simulink model "HEV"  (R2015a)
settings: Solver=ode23tb  StartTime=0.0  StopTime=318  FixedStep=Ts  MaxStep=Ts  RelTol=1  AbsTol=0.5
InitFcn:
  | Ts = 6e-05;   % time step
  | DriveCycleNumber = 1;
  | beginningSim = 1;
undefined symbols (not defined in the file): drive_block, drive_enginemodel, EngineSpeedPower, FuelConsTable, GasEmisTable, h, Hydride, km, magnitude, Metal, Nickel, rad, s, speed, torque
libraries: powerlib x47, driveline x30, simulink x13, simulink_extras x9, electricdrivelib x3, powerlib_extras x3, aerolibconvert2 x2, DC6DriveInternalModels x1
(part 1 of 3)
settings Model: SimulationMode=accelerator  TunableVars=EngineSpeedPower,FuelConsTable,GasEmisTable,ftp75,nedc  TunableVarsStorageClass=Auto,Auto,Auto,Auto,Auto  TunableVarsTypeQualifier=,,,,  Creator=Elena  LastModifiedBy=Elena
settings SolverCC: MaxConsecutiveMinStep=10000  ZeroCrossControl=DisableAll
settings DataIOCC: SaveCompleteFinalSimState=on  SaveFormat=Dataset
settings OptimizationCC: InlineParams=on
settings DebuggingCC: UnderspecifiedInitializationDetection=Classic  SignalResolutionControl=TryResolveAllWithWarning  SigSpecEnsureSampleTimeMsg=none  FcnCallInpInsideContextMsg=UseLocalSettings
settings SimscapeCC: SimscapeLogSimulationStatistics=on

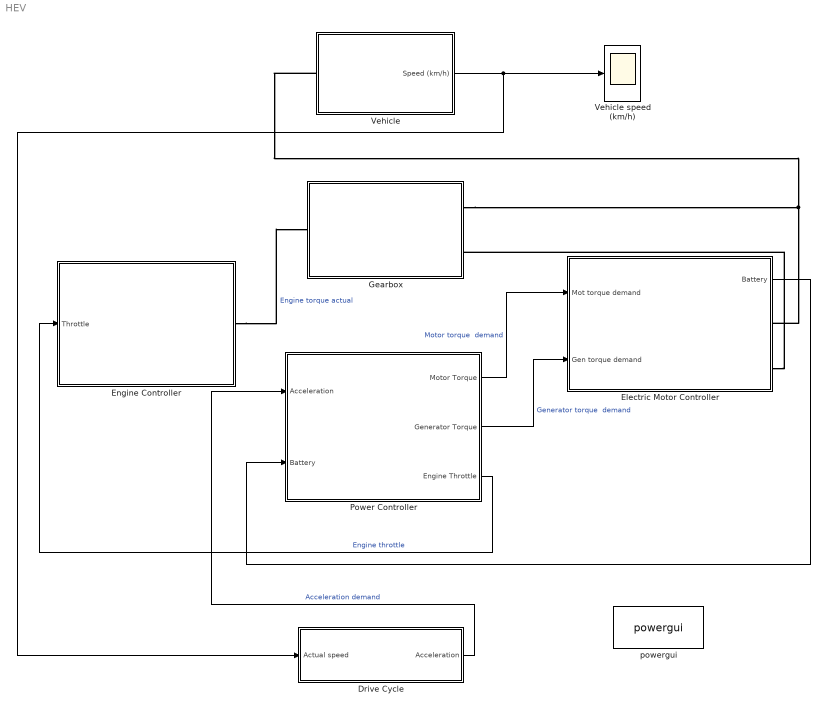
== system HEV ==
  Drive Cycle : Subsystem
  "Electric Motor Controller " : Subsystem
  Engine Controller : Subsystem
  Gearbox : Subsystem
  Power Controller : Subsystem
  Vehicle : Subsystem
  Vehicle speed (km/h) : Scope
      settings: YMin=25.2384  YMax=25.2387  SaveName=ScopeData4  Decimation=10
  powergui : powerlib/powergui  SimulationMode=Discrete  SolverType=Tustin  SampleTime=Ts  frequency=60  SPID=on  DisableSnubberDevices=off  DisableRonSwitches=off  DisableVfSwitches=off  SwTol=0  DisplayEquations=off  Interpol=off  methode=off  Ts=0  FunctionMessages=off  echomessages=off  HookPort=off  EnableUseOfTLC=off  x0status=blocks  frequencyindice=0  Pbase=100e6  ErrMax=1e-4  Iterations=50  UnitsV=kV  UnitsW=MW  buscounter=0  RestoreLinks=warning  ResistiveCurrentMeasurement=off  Frange=[0:2:500]  Ylog=off  Xlog=on  ShowGrid=off  save=off  variable=ZData  structure=0  ZoomFFT=on  StartTime=0.0  cycles=1  DisplayStyle=1  fundamental=60  FreqAxis=off  MaxFrequency=1000  frequencyindicesteady=1  RmsSteady=1  display=off
  wires:
  Power Controller/3(Engine Throttle) -> Engine Controller/1(Throttle)  "Engine throttle"
  Vehicle/1(Speed (km/h)) -> Drive Cycle/1(Actual speed), Vehicle speed (km/h)/1
  Drive Cycle/1("Acceleration ") -> Power Controller/1(Acceleration)  "Acceleration demand"
  "Electric Motor Controller "/1(Battery) -> Power Controller/2(Battery)
  Power Controller/1(Motor Torque) -> "Electric Motor Controller "/1(Mot torque demand)  "Motor torque  demand"
  Power Controller/2(Generator Torque) -> "Electric Motor Controller "/2("Gen torque demand ")  "Generator torque  demand"
  connections:
  Engine Controller/RConn1 -- Gearbox/LConn1  "Engine torque actual"
  Vehicle/LConn1 -- Gearbox/RConn1 -- "Electric Motor Controller "/RConn1
  "Electric Motor Controller "/RConn2 -- Gearbox/RConn2

== system HEV/Drive Cycle ==
  Actual speed : Inport
  Actual speed. : Display
      settings: Decimation=100
  Constant : Constant  Value=final_actualSpeed(end)
  Constant1 : Constant  Value=beginningSim
  Control : Constant  Value=DriveCycleNumber
  Demanded speed : Display
      settings: Decimation=100
  FTP75 : FromWorkspace  VariableName=[ftp75_1.seconds ftp75_1.kph]  SampleTime=0
  Multiport Switch : MultiPortSwitch  Inputs=2
  NEDC : FromWorkspace  VariableName=[nedc.seconds nedc.kph]  SampleTime=0
  Speed Control : Subsystem
  Switch : Switch  Criteria=u2 ~= 0
  To Workspace : ToWorkspace  VariableName=final_actualSpeed  SampleTime=20
      settings: Save2DSignal=2-D array (concatenate along first dimension)
  "Acceleration " : Outport
  wires:
  Control/1 -> Multiport Switch/1
  FTP75/1 -> Multiport Switch/2
  NEDC/1 -> Multiport Switch/3
  Multiport Switch/1 -> Demanded speed/1, Speed Control/1(Demanded speed)
  Speed Control/1(Acceleration) -> "Acceleration "/1
  Constant/1 -> Switch/3
  Actual speed/1 -> Switch/1
  Constant1/1 -> Switch/2
  Switch/1 -> To Workspace/1, Actual speed./1, Speed Control/2(Actual speed)

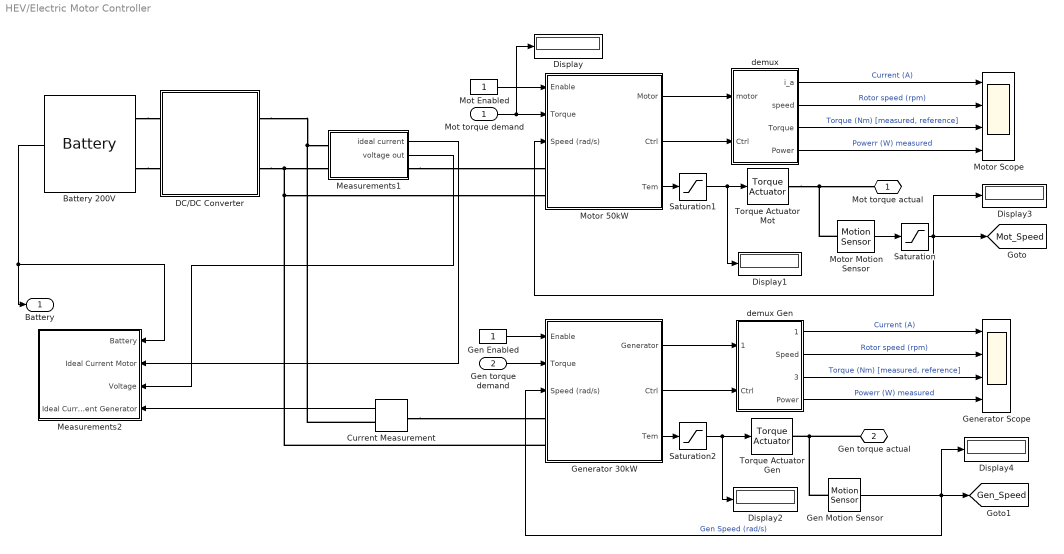
== system HEV/Electric Motor Controller  ==
  Mot torque demand : Inport
  "Gen torque demand " : Inport  Port=2
  Battery 200V : electricdrivelib/Extra Sources/Battery  BatType=Nickel-Metal-Hydride  ShowDetailedParameters=off  NomV=200  NomQ=6.5  SOC=final_SOC(end)  PresetModel=on  MaxQ=7  FullV=235.5932  Dis_rate=1.3  R=0.30769  Normal_OP=6.25  expZone="[216.9492           1.3]"  current=[50 100]  Units=Time  Batt_Tr=30
  Current Measurement : powerlib/Measurements/Current Measurement  PhasorSimulation=off  OutputType=Complex  PSBequivalent=0
  DC/DC Converter : Subsystem
      mask init:
      | [X1,X1m,X2,X2m,X3,X4,Y1,Y1m,Y2,Y2m,Y3,Y4,color1,color2]=spsdrivelogo;
      mask Display:
      | patch([X1 X1m],[Y1 Y1m],color1);
      | patch(X3,Y3,color2);
      | plot([X1 X1m X2 X2m X3 X4],[Y1 Y1m Y2 Y2m Y3 Y4]);
  Display{,1..4} (5 alike) : Display
      settings: Decimation=100
  Gen Enabled : Constant
  Gen Motion Sensor : driveline/Sensors & Actuators/Motion Sensor  Angle=off  x0=0  Velocity=on  Acceleration=off
  Generator 30kW : Subsystem
  Generator Scope : Scope  NumInputPorts=4
      settings: TimeRange=320  YMin=-125~-750~-0.045~-2.5  YMax=125~1500~0.015~1  Decimation=100
  Measurements1 : Subsystem
  Measurements2 : Subsystem
  Mot Enabled : Constant
  Motor 50kW : Subsystem
  Motor Motion Sensor : driveline/Sensors & Actuators/Motion Sensor  Angle=off  x0=0  Velocity=on  Acceleration=off
  Motor Scope : Scope  NumInputPorts=4
      settings: TimeRange=320  YMin=-500~1505.5~-175~3915  YMax=400~1508.25~125~3970  Decimation=100
  Saturation : Saturate  UpperLimit=6000*pi/30  LowerLimit=0
  Saturation1 : Saturate  UpperLimit=400  LowerLimit=-400
  Saturation2 : Saturate  UpperLimit=400  LowerLimit=-400
  Torque Actuator Gen : driveline/Sensors & Actuators/Torque Actuator
  Torque Actuator Mot : driveline/Sensors & Actuators/Torque Actuator
  demux : Subsystem
  demux Gen : Subsystem
  Mot torque actual : PMIOPort  Port=1  Side=Right
  Gen torque actual : PMIOPort  Port=2  Side=Right
  Battery : Outport
  tag scope: Gen_Speed=global, Mot_Speed=global
  wires:
  Battery 200V/1 -> Measurements2/1(Battery), Battery/1
  Mot Enabled/1 -> Motor 50kW/1(Enable)
  Mot torque demand/1 -> Display/1, Motor 50kW/2(Torque)
  "Gen torque demand "/1 -> Generator 30kW/2(Torque)
  Gen Enabled/1 -> Generator 30kW/1(Enable)
  Motor 50kW/1(Motor) -> demux/1(motor)
  Motor 50kW/3(Tem) -> Saturation1/1
  Generator 30kW/3(Tem) -> Saturation2/1
  demux/1(i_a) -> Motor Scope/1  "Current (A)"
  demux/2(speed) -> Motor Scope/2  "Rotor speed (rpm)"
  demux/3(Torque) -> Motor Scope/3  "Torque (Nm) [measured, reference]"
  Generator 30kW/2(Ctrl) -> demux Gen/2(Ctrl)
  Generator 30kW/1(Generator) -> demux Gen/1(Generator)
  demux Gen/1(Current) -> Generator Scope/1  "Current (A)"
  demux Gen/2(Speed) -> Generator Scope/2  "Rotor speed (rpm)"
  demux Gen/3(Torque) -> Generator Scope/3  "Torque (Nm) [measured, reference]"
  demux Gen/4(Power) -> Generator Scope/4  "Powerr (W) measured"
  Measurements1/1(" ideal current ") -> Measurements2/2(Ideal Current Motor)
  Current Measurement/1 -> Measurements2/4(Ideal Current Generator)
  Gen Motion Sensor/1 -> Display4/1, Generator 30kW/3(Speed (rad/s)), [Gen_Speed]  "Gen Speed (rad/s)"
  Motor 50kW/2(Ctrl) -> demux/2(Ctrl)
  Measurements1/2(voltage out) -> Measurements2/3(Voltage)
  Motor Motion Sensor/1 -> Saturation/1
  Saturation1/1 -> Display1/1, Torque Actuator Mot/1
  Saturation2/1 -> Display2/1, Torque Actuator Gen/1
  Saturation/1 -> Display3/1, [Mot_Speed], Motor 50kW/3(Speed (rad/s))
  demux/4(Power) -> Motor Scope/4  "Powerr (W) measured"
  connections:
  Battery 200V/LConn1 -- DC/DC Converter/LConn1
  Battery 200V/LConn2 -- DC/DC Converter/LConn2
  Generator 30kW/LConn2 -- DC/DC Converter/RConn2 -- Measurements1/LConn2 -- Motor 50kW/LConn2
  Current Measurement/RConn1 -- DC/DC Converter/RConn1 -- Measurements1/LConn1
  Measurements1/RConn1 -- Motor 50kW/LConn1
  Current Measurement/LConn1 -- Generator 30kW/LConn1
  Gen torque actual/RConn1 -- Gen Motion Sensor/LConn1 -- Torque Actuator Gen/RConn1
  Torque Actuator Mot/RConn1 -- Motor Motion Sensor/LConn1 -- Mot torque actual/RConn1

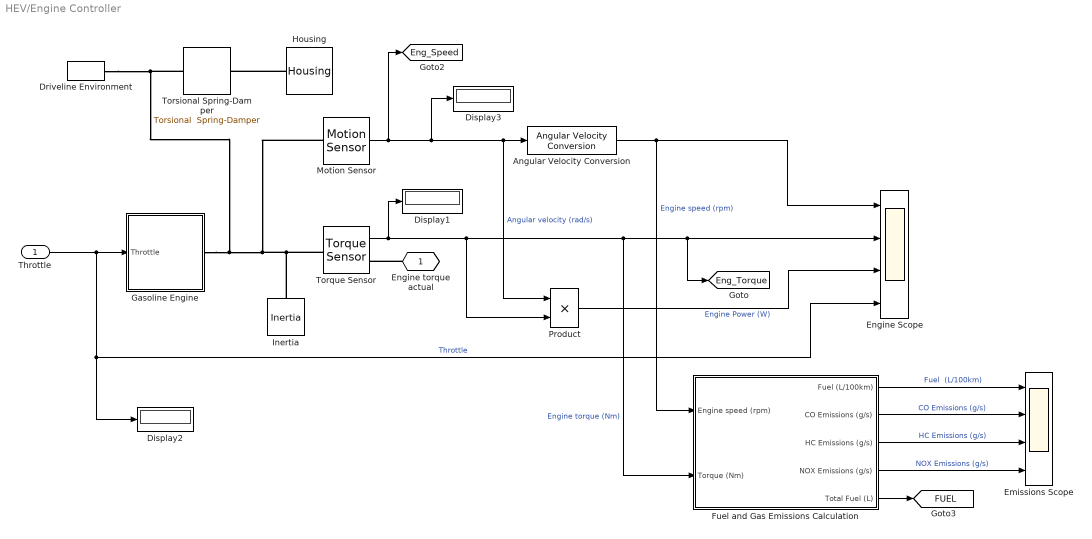
== system HEV/Engine Controller ==
  Throttle : Inport
  Angular Velocity Conversion : aerolibconvert2/Angular Velocity Conversion  IU=rad/s  OU=rpm
  Display1 : Display
      settings: Decimation=100
  Display2 : Display
  Display3 : Display
      settings: Decimation=100
  Driveline Environment : driveline/Solver & Inertias/Driveline Environment  PortType=p1  BlockClass=Solver  PhysicalDomain=driveline_domain  SimulationMode=Dynamics  ModeIteration=on  DefaultClutchVelocityTolerance=1e-3  DefaultUseAutoClutchVelocityTolerance=off
  Emissions Scope : Scope  NumInputPorts=4
      settings: TimeRange=157  YMin=-500~0.187868~0.0455781~-1  YMax=3500~0.187868~0.0455781~1  SaveName=ScopeData5  Decimation=100
  Engine Scope : Scope  NumInputPorts=4
      settings: TimeRange=320  YMin=-500~0~0~-1  YMax=3500~130~800~1  SaveName=ScopeData7  Decimation=100
  Fuel and Gas Emissions Calculation : Subsystem
  Gasoline Engine : Subsystem  AncestorBlock=driveline/Vehicle Components/Gasoline Engine  DialogController=PMDialogs.PMDefaultMaskDlg  LoadFcn=drive_block('LoadFcn');  StartFcn=drive_enginemodel('Start');  mask(Gasoline Engine){power_max=57000, speed_at_power_max=5000, speed_max=6000}
      mask prompts: power_max "Maximum power [W]:"; speed_at_power_max "Speed at maximum power [rpm]:"; speed_max "Maximum speed [rpm]:"
      mask help:
      | Simple gasoline fuel engine model with speed governor.  The throttle input signal lies between zero and one and specifies the torque demanded from the engine as a fraction of the maximum possible torque.  This signal also indirectly controls the engine speed.  The engine model does not include air-fuel combustion dynamics.
      |
      | If the throttle signal rises above one or falls below zero, the engine limits the signal to one or zero, respectively. If the engine speed rises above the maximum speed, the engine torque drops to zero.
      mask init:
      | drive_preinitmask();[speed,power,torque,p] = ...
      | 	drive_enginemodel('MaskGasoline');
      settings: CopyFcn=drive_block('CopyFcn');  DeleteFcn=drive_block('DeleteFcn');  ModelCloseFcn=drive_block('ModelCloseFcn');  PreSaveFcn=drive_block('PreSaveFcn');  PostSaveFcn=drive_block('PostSaveFcn');  PreCopyFcn=drive_block('PreCopyFcn');  PreDeleteFcn=drive_block('PreDeleteFcn');
      mask Help: web(drive_help);
      mask Display:
      | image(imread('engine.bmp'),'center')
      | plot(speed, torque/max(torque))
      | plot(speed, power/max(power))
      | port_label('input', 1, 'Throttle')
  Housing : driveline/Solver & Inertias/Housing
  Inertia : driveline/Solver & Inertias/Inertia  PortType=p1  BlockClass=Inertia  PhysicalDomain=driveline_domain  I=0.25  Ip=[]  Iv=[]  ShowLeft=off  ShowRight=on
  Motion Sensor : driveline/Sensors & Actuators/Motion Sensor  Angle=off  x0=0  Velocity=on  Acceleration=off
  Product : Product
  Torque Sensor : driveline/Sensors & Actuators/Torque Sensor
  Torsional Spring-Damper : driveline/Dynamic Elements/Torsional  Spring-Damper  k=0  c=0.2079  x0=0  Backlash=0
  Engine torque actual : PMIOPort  Port=1  Side=Right
  tag scope: Eng_Speed=global, Eng_Torque=global, FUEL=global
  wires:
  Throttle/1 -> Display2/1, Engine Scope/4, Gasoline Engine/1(Throttle)  "Throttle"
  Motion Sensor/1 -> [Eng_Speed], Display3/1, Angular Velocity Conversion/1, Product/1  "Angular velocity (rad/s)"
  Angular Velocity Conversion/1 -> Fuel and Gas Emissions Calculation/1(Engine speed (rpm)), Engine Scope/1  "Engine speed (rpm)"
  Torque Sensor/1 -> Display1/1, Fuel and Gas Emissions Calculation/2(Torque (Nm)), Engine Scope/2, [Eng_Torque], Product/2  "Engine torque (Nm)"
  Product/1 -> Engine Scope/3  "Engine Power (W)"
  Fuel and Gas Emissions Calculation/1(Fuel (L/100km)) -> Emissions Scope/1  "Fuel  (L/100km)"
  Fuel and Gas Emissions Calculation/2(CO Emissions (g/s)) -> Emissions Scope/2  "CO Emissions (g/s)"
  Fuel and Gas Emissions Calculation/3(HC Emissions (g/s)) -> Emissions Scope/3  "HC Emissions (g/s)"
  Fuel and Gas Emissions Calculation/4(NOX Emissions (g/s)) -> Emissions Scope/4  "NOX Emissions (g/s)"
  Fuel and Gas Emissions Calculation/5(Total Fuel (L)) -> [FUEL]
  connections:
  Motion Sensor/LConn1 -- Driveline Environment/LConn1 -- Torsional Spring-Damper/LConn1 -- Gasoline Engine/RConn1 -- Inertia/RConn1 -- Torque Sensor/LConn1
  Housing/RConn1 -- Torsional Spring-Damper/RConn1
  Engine torque actual/RConn1 -- Torque Sensor/RConn1

== system HEV/Gearbox ==
  Add3 : Sum
  Eng Motion Sensor : driveline/Sensors & Actuators/Motion Sensor  Angle=off  x0=0  Velocity=on  Acceleration=off
  Gen Motion Sensor : driveline/Sensors & Actuators/Motion Sensor  Angle=off  x0=0  Velocity=on  Acceleration=off
  Mot Motion Sensor : driveline/Sensors & Actuators/Motion Sensor  Angle=off  x0=0  Velocity=on  Acceleration=off
  Mux2 : Mux  Inputs=2
  Planetary Gear : driveline/Gears/Planetary Gear  Ratio=2.6  Show=off  LinearizationFlag=off  ValidatorFcn=drive_planetarygearblock
  Power (w) : Scope  NumInputPorts=3
      settings: YMin=-2500~-1000~-2500  YMax=32500~12000~22500  SaveName=ScopeData9  Decimation=100
  Product : Product  RndMeth=Zero
  Product1 : Product  RndMeth=Zero
  Product2 : Product  RndMeth=Zero
  Speed (rad/s) : Scope  NumInputPorts=3
      settings: YMin=5.775e+81~-1.516e+82~-4.5e+68  YMax=6.175e+81~-1.503e+82~5e+67  SaveName=ScopeData3  Decimation=100
  Torque (Nm) : Scope  NumInputPorts=3
      settings: YMin=-10~-5~-2.5  YMax=130~90~35  SaveName=ScopeData10  Decimation=100
  Torque Sensor1 : driveline/Sensors & Actuators/Torque Sensor
  Torque Sensor2 : driveline/Sensors & Actuators/Torque Sensor
  Torque Sensor3 : driveline/Sensors & Actuators/Torque Sensor
  Engine Torque : PMIOPort  Port=1  Side=Left
  Motor Torque : PMIOPort  Port=2  Side=Right
  Generator Torque : PMIOPort  Port=3  Side=Right
  wires:
  Eng Motion Sensor/1 -> Speed (rad/s)/3, Product/1  "Carrier speed (rad/s) - Engine"
  Gen Motion Sensor/1 -> Speed (rad/s)/2, Product2/1  "Sun speed (rad/s) - Generator"
  Mot Motion Sensor/1 -> Speed (rad/s)/1, Product1/2  "Ring speed (rad/s) - Motor"
  Torque Sensor1/1 -> Product/2, Torque (Nm)/1  "Carrier torque (Nm) - Engine"
  Torque Sensor3/1 -> Torque (Nm)/3, Product2/2  "Sun torque (Nm) - Generator"
  Torque Sensor2/1 -> Torque (Nm)/2, Product1/1  "Ring torque (Nm) - Motor"
  Add3/1 -> Mux2/2
  Product/1 -> Mux2/1
  Product1/1 -> Power (w)/3, Add3/1  "Ring power (W) - Motor"
  Product2/1 -> Power (w)/2, Add3/2  "Sun power (W) - Generator"
  Mux2/1 -> Power (w)/1  "Carrier power (W) - Engine"
  connections:
  Torque Sensor2/LConn1 -- Planetary Gear/RConn1
  Eng Motion Sensor/LConn1 -- Planetary Gear/LConn1 -- Torque Sensor1/RConn1
  Torque Sensor1/LConn1 -- Engine Torque/RConn1
  Torque Sensor2/RConn1 -- Mot Motion Sensor/LConn1 -- Motor Torque/RConn1
  Torque Sensor3/RConn1 -- Gen Motion Sensor/LConn1 -- Generator Torque/RConn1
  Torque Sensor3/LConn1 -- Planetary Gear/RConn2

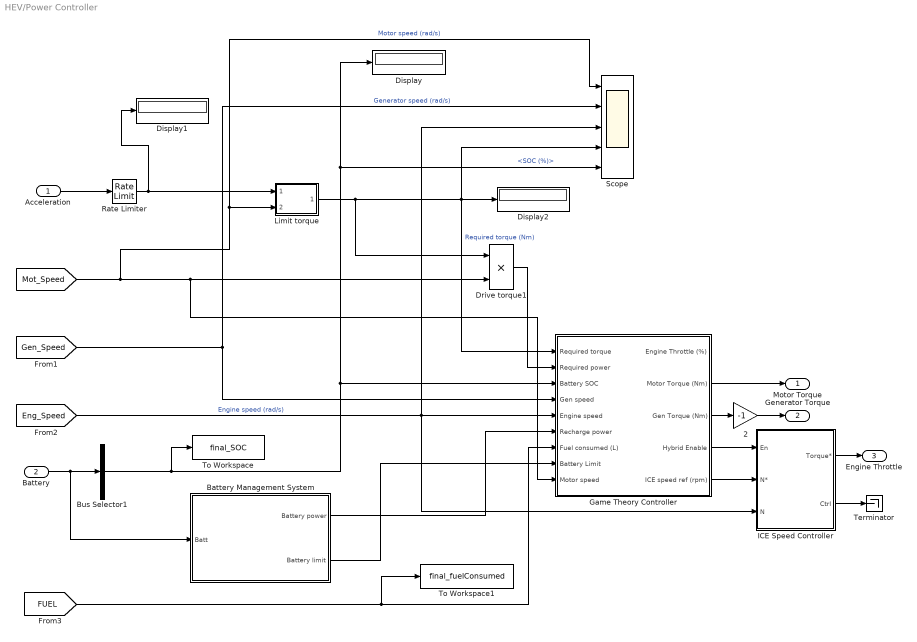
== system HEV/Power Controller ==
  Acceleration : Inport
  Battery : Inport  Port=2
  " 2" : Gain  Gain=-1
  Battery Management System : Subsystem
      mask init:
      | [X1,X1m,X2,X2m,X3,X4,Y1,Y1m,Y2,Y2m,Y3,Y4,color1,color2]=spsdrivelogo;
      mask Display:
      | patch([X1 X1m],[Y1 Y1m],color1);
      | patch(X3,Y3,color2);
      | plot([X1 X1m X2 X2m X3 X4],[Y1 Y1m Y2 Y2m Y3 Y4]);
  Bus Selector1 : BusSelector  OutputSignals=SOC (%)
  Display : Display
      settings: Decimation=100
  Display1 : Display
      settings: Decimation=100
  Display2 : Display
      settings: Decimation=100
  Drive torque1 : Product  Inputs=**  OutDataTypeStr=double
  Game Theory Controller : Subsystem
  ICE Speed Controller : Subsystem  mask(Speed controller){SwK=Speed regulation, bs=1800, ramp=[-5000,5000]*10, kp=0.01, ki=0.1, fc=100, ctrl_sat=[0,1], Tsc=Ts}
      mask prompts: SwK "Regulation type"; bs "Base speed (rpm)"; ramp "Speed reference ramp (rpm/s) [deceleration,acceleration]"; kp "Proportional gain"; ki "Integral gain"; fc "Speed measurement - low-pass filter cutoff frequency (Hz)"; ctrl_sat "Controller output torque saturation (N.m) [negative,positive]"; Tsc "Controller sampling time (s)"
      mask help: This block implements a PI speed regulator.
      mask init:
      | [X1,X1m,X2,X2m,X3,X4,Y1,Y1m,Y2,Y2m,Y3,Y4,color1,color2]=spsdrivelogo;
      mask TypeOptions SwK: Speed regulation | Torque regulation
      mask Display:
      | patch([X1 X1m],[Y1 Y1m],color1);
      | patch(X3,Y3,color2);
      | plot([X1 X1m X2 X2m X3 X4],[Y1 Y1m Y2 Y2m Y3 Y4]);
  Limit torque : Subsystem
      mask Display: plot([0;1800;2000;2500;3000;3500], [1;1;0.90*1;0.72*1;0.6*1;0.51*1])
  Rate Limiter : RateLimiter  SampleTimeMode=inherited
  Scope : Scope  NumInputPorts=5
      settings: TimeRange=318  YMin=0~-750~-50~114~32.5  YMax=350~750~350~122~55  SaveName=ScopeData8  Decimation=100
  Terminator : Terminator
  To Workspace : ToWorkspace  VariableName=final_SOC  SampleTime=20
      settings: Save2DSignal=2-D array (concatenate along first dimension)
  To Workspace1 : ToWorkspace  VariableName=final_fuelConsumed  SampleTime=20
      settings: Save2DSignal=2-D array (concatenate along first dimension)
  Motor Torque : Outport
  Generator Torque : Outport  Port=2
  Engine Throttle : Outport  Port=3
  wires:
  Acceleration/1 -> Rate Limiter/1
  Rate Limiter/1 -> Limit torque/1(Acceleration), Display1/1
  [Mot_Speed] -> Game Theory Controller/9(Motor speed), Drive torque1/2, Limit torque/2(Motor Speed (rad/s)), Scope/1  "Motor speed (rad/s)"
  Limit torque/1(torque) -> Game Theory Controller/1(Required torque), Display2/1, Scope/4, Drive torque1/1  "Required torque (Nm)"
  [Gen_Speed] -> Scope/2, Game Theory Controller/4(Gen speed)  "Generator speed (rad/s)"
  [Eng_Speed] -> Scope/3, Game Theory Controller/5(Engine speed), ICE Speed Controller/3(N)  "Engine speed (rad/s)"
  Game Theory Controller/2(Motor Torque (Nm)) -> Motor Torque/1
  Battery/1 -> Battery Management System/1(Batt), Bus Selector1/1
  Bus Selector1/1 -> To Workspace/1, Display/1, Scope/5, Game Theory Controller/3(Battery SOC)  "<SOC (%)>"
  Battery Management System/1(Battery power) -> Game Theory Controller/6(Recharge power)
  [FUEL] -> To Workspace1/1, Game Theory Controller/7(Fuel consumed (L))
  Drive torque1/1 -> Game Theory Controller/2(Required power)
  Game Theory Controller/3(Gen Torque (Nm)) -> " 2"/1
  " 2"/1 -> Generator Torque/1
  Game Theory Controller/5(ICE speed ref (rpm)) -> ICE Speed Controller/2(N*)
  Game Theory Controller/4(Hybrid Enable) -> ICE Speed Controller/1(En)
  ICE Speed Controller/2(Ctrl) -> Terminator/1
  Battery Management System/2(Battery limit) -> Game Theory Controller/8(Battery Limit)
  ICE Speed Controller/1(Torque*) -> Engine Throttle/1

== system HEV/Vehicle ==
  Differential : driveline/Gears/Differential  R=1  ValidatorFcn=drive_differentialgearblock  SimDrivelineLibraryVersion=1.1
  Display : Display
      settings: Decimation=100
  Housing : driveline/Solver & Inertias/Housing
  Incline angle : Constant  Value=0
  Left Tire : driveline/Vehicle Components/Tire  r_e=0.3  F_z=3000  F_x_max=3500  kappa_max=10  sigma_k=0.2
  Left Tire Inertia : driveline/Solver & Inertias/Inertia  PortType=p1  BlockClass=Inertia  PhysicalDomain=driveline_domain  I=0.5  Ip=[]  Iv=[]  ShowLeft=off  ShowRight=on
  Longitudinal Vehicle Dynamics : driveline/Vehicle Components/Longitudinal Vehicle Dynamics  m=1325  a=1.35  b=1.35  h=0.5  FA=2.57  C_d=0.26  v0=0
  Right Tire : driveline/Vehicle Components/Tire  r_e=0.3  F_z=3000  F_x_max=3500  kappa_max=10  sigma_k=0.2
  Right Tire Inertia : driveline/Solver & Inertias/Inertia  PortType=p1  BlockClass=Inertia  PhysicalDomain=driveline_domain  I=0.5  Ip=[]  Iv=[]  ShowLeft=off  ShowRight=on
  Saturation : Saturate  UpperLimit=200  LowerLimit=0
  Simple Gear : driveline/Gears/Simple Gear  PortType=p1  BlockClass=SimpleGear  PhysicalDomain=driveline_domain  Reversing=off  Ratio=4.113
  Terminator1 : Terminator
  Terminator2 : Terminator
  Torque Sensor : driveline/Sensors & Actuators/Torque Sensor
  Torsional Spring-Damper (Friction) : driveline/Dynamic Elements/Torsional  Spring-Damper  k=0  c=0.1  x0=0  Backlash=0
  Transmission Inertia : driveline/Solver & Inertias/Inertia  PortType=p1  BlockClass=Inertia  PhysicalDomain=driveline_domain  I=0.5  Ip=[]  Iv=[]  ShowLeft=off  ShowRight=on
  m/s to km/h : Gain  Gain=(60*60)/1000
  Torque : PMIOPort  Port=1  Side=Left
  Speed (km/h) : Outport
  tag scope: VehSpeed_kmh=global
  wires:
  Left Tire/2 -> Longitudinal Vehicle Dynamics/1
  Right Tire/2 -> Longitudinal Vehicle Dynamics/2
  Incline angle/1 -> Longitudinal Vehicle Dynamics/3
  Longitudinal Vehicle Dynamics/3 -> Right Tire/2
  Longitudinal Vehicle Dynamics/2 -> Left Tire/2
  Longitudinal Vehicle Dynamics/1 -> m/s to km/h/1, Right Tire/1, Left Tire/1
  Left Tire/1 -> Terminator1/1
  Right Tire/1 -> Terminator2/1
  Torque Sensor/1 -> Display/1
  m/s to km/h/1 -> Saturation/1
  Saturation/1 -> [VehSpeed_kmh], Speed (km/h)/1
  connections:
  Torque Sensor/LConn1 -- Torque/RConn1
  Torsional Spring-Damper (Friction)/RConn1 -- Simple Gear/LConn1 -- Torque Sensor/RConn1
  Housing/RConn1 -- Torsional Spring-Damper (Friction)/LConn1
  Simple Gear/RConn1 -- Transmission Inertia/RConn1 -- Differential/LConn1
  Left Tire Inertia/RConn1 -- Left Tire/LConn1 -- Differential/RConn1
  Right Tire Inertia/RConn1 -- Right Tire/LConn1 -- Differential/RConn2

== system HEV/Drive Cycle/Speed Control ==
  Demanded speed : Inport
  Actual speed : Inport  Port=2
  Display : Display
      settings: Decimation=100
  Display1 : Display
      settings: Decimation=100
  Display2 : Display
      settings: Decimation=100
  Integrator [-5,5] : Integrator  LimitOutput=on  UpperSaturationLimit=5  LowerSaturationLimit=-5
  Ki : Gain  Gain=0.04
  Kp : Gain  Gain=0.02
  Limit : Saturate  UpperLimit=1  LowerLimit=-1
  Lowpass Filter 20Hz : TransferFcn  Denominator=[1/(2*pi*20) 1]
  Mux : Mux  Inputs=2
  Scope : Scope  NumInputPorts=2
      settings: TimeRange=318  YMin=86.25~0.289  YMax=88.75~0.303  SaveName=ScopeData6  Decimation=100
  Sum1 : Sum  Inputs=++|
  Sum2 : Sum  Inputs=+-|
  Acceleration : Outport
  wires:
  Limit/1 -> Display2/1, Acceleration/1, Scope/2  "Acceleration"
  Demanded speed/1 -> Mux/2, Display1/1, Sum2/1  "Demanded speed"
  Actual speed/1 -> Mux/1, Lowpass Filter 20Hz/1  "Actual speed"
  Sum1/1 -> Limit/1
  Ki/1 -> Integrator [-5,5]/1
  Kp/1 -> Sum1/1
  Integrator [-5,5]/1 -> Sum1/2
  Lowpass Filter 20Hz/1 -> Display/1, Sum2/2
  Sum2/1 -> Ki/1, Kp/1
  Mux/1 -> Scope/1  "Speed km/h [actual, reference]"

== system HEV/Electric Motor Controller /DC//DC Converter ==
  Bus DC controller : Subsystem
  DC/DC converter : Subsystem
  Ubus Ref : Constant  Value=500
  +Vdc Bus : PMIOPort  Tag=PMCPort  Port=1  Side=Right
  -Vdc Bus : PMIOPort  Tag=PMCPort  Port=2  Side=Right
  + battery : PMIOPort  Tag=PMCPort  Port=3  Side=Left
  - battery : PMIOPort  Tag=PMCPort  Port=4  Side=Left
  wires:
  Ubus Ref/1 -> Bus DC controller/2(Uref)
  Bus DC controller/1(Duty cycle) -> DC/DC converter/1(Duty Cycle)
  DC/DC converter/1(UBus) -> Bus DC controller/1(Ubus)
  connections:
  +Vdc Bus/RConn1 -- DC/DC converter/LConn1
  -Vdc Bus/RConn1 -- DC/DC converter/LConn2
  + battery/RConn1 -- DC/DC converter/RConn1
  - battery/RConn1 -- DC/DC converter/RConn2

== system HEV/Electric Motor Controller /Generator 30kW ==
  Enable : Inport
  Torque : Inport  Port=2
  Speed (rad/s) : Inport  Port=3
  Bus Selector : BusSelector  OutputSignals=Rotor speed wm (rad/s),Rotor angle thetam (rad),Electromagnetic torque Te (N*m)
  Measures : electricdrivelib/AC drives/PM Synchronous Motor Drive/Measures
  Mux : Subsystem
  PMSM1 : powerlib/Machines/Permanent Magnet Synchronous Machine  NbPhases=3  FluxDistribution=Sinusoidal  RotorType=Salient-pole  MechanicalLoad=Speed w  PresetModel=No  ShowDetailedParameters=on  MeasurementBus=off  Resistance=0.05  Inductance=0  dqInductances=[0.000635 0.000635]  La=0.000835  MachineConstant=Flux linkage established by magnets (V.s)  Flux=0.192  VoltageCst=34.8249  TorqueCst=0.288  Flat=0  Mechanical=[0.011 0.001889/4 4/4]  PolePairs=1  InitialConditions=[0,0, 0,0,0]  InitialConditions5ph=[0 0 0 0 0 0]  TsPowergui=0  TsBlock=-1  RefAngle=90 degrees behind phase A axis (modified Park)
      settings: AttributesFormatString=\n
  Speed Controller : Subsystem  mask(Speed controller){SwK=Torque regulation, bs=1800, ramp=[-5000,5000], kp=(1/5)/4, ki=(50/5)/4/3, fc=(1000/10)/2, ctrl_sat=[-45,45], Tsc=Ts}
      mask prompts: SwK "Regulation type"; bs "Base speed (rpm)"; ramp "Speed reference ramp (rpm/s) [deceleration,acceleration]"; kp "Proportional gain"; ki "Integral gain"; fc "Speed measurement - low-pass filter cutoff frequency (Hz)"; ctrl_sat "Controller output torque saturation (N.m) [negative,positive]"; Tsc "Controller sampling time (s)"
      mask help: This block implements a PI speed regulator.
      mask init:
      | [X1,X1m,X2,X2m,X3,X4,Y1,Y1m,Y2,Y2m,Y3,Y4,color1,color2]=spsdrivelogo;
      mask TypeOptions SwK: Speed regulation | Torque regulation
      mask Display:
      | patch([X1 X1m],[Y1 Y1m],color1);
      | patch(X3,Y3,color2);
      | plot([X1 X1m X2 X2m X3 X4],[Y1 Y1m Y2 Y2m Y3 Y4]);
  Three-phase Inverter : Subsystem  mask(SPSdrives Converter){Arms=3, SnubberResistance=5000, SnubberCapacitance=inf, Device=IGBT / Diodes, Ron=1e-3, Lon=0, ForwardVoltages=[0.8,0.8], ForwardVoltage=0, GTOparameters=[0,0], IGBTparameters=[1e-6,2e-6], Measurements=All voltages and currents, SourceFrequency=60, dqInductances=[0.000635,0.000635], Flux=0.192, Resistance=0.05, p=4/4, converterType=Inverter}
      mask prompts: Arms "Number of bridge arms:"; SnubberResistance "Snubber resistance Rs (Ohms)"; SnubberCapacitance "Snubber capacitance Cs (F)"; Device "Power Electronic device"; Ron "Ron (Ohms)"; Lon "Lon (H)"; ForwardVoltages "Forward voltages  [ Device Vf(V) , Diode Vfd(V)]"; ForwardVoltage "Forward voltage Vf (V)"; GTOparameters "[  Tf (s) , Tt (s)  ]"; IGBTparameters "[  Tf (s) , Tt (s)  ]"; SourceFrequency "Source Frequency (Hz)"; dqInductances "PMSM-Inductances [ Ld(H) Lq(H) ]:"; Flux "PMSM-Flux induced by magnets (Wb):"; Resistance "PMSM-Stator resistance Rs (ohm):"; p "PMSM-Pairs of poles p:"; converterType "Converter type:"
      mask init:
      | Ld=dqInductances(1);
      | Lq=dqInductances(2);
      | Fcs=6*SourceFrequency/10;
      settings: OpenFcn=power_openblockproxy();
      mask Help: web(psbhelp);
      mask TypeOptions Arms: 1 | 2 | 3
      mask TypeOptions Device: Diodes | Thyristors | GTO / Diodes | MOSFET / Diodes | IGBT / Diodes | Ideal Switches
      mask TypeOptions Measurements: None | Device voltages | Device currents | UAB UBC UCA UDC voltages | All voltages and currents
      mask TypeOptions converterType: Rectifier | Inverter
      mask Display: plot(0,0,100,100,[39 39 23.8],[71 28 28],[44 56 49.6 56 52.8 56 61 61],[39.2 33.6 32.8 33.6 40.8 33.6 30 12.4],[44 44 44 61 61],[28 71 60 66.4 90],[75 67 83 75 67 83 75 75],[54 42 42 54 54 54 54 66],[61 75 75],[24 24 42],[75 75 61],[66,76,76])
  VECT : Subsystem  mask(VECT){nb_p=4/4, lambda=0.192, freq_max=20e3, Ts_vect=Ts, h=2}
      mask prompts: nb_p "Motor pairs of poles"; lambda "Flux induced by magnets (Wb)"; freq_max "Maximum switching frequency (Hz)"; Ts_vect "Sampling time (s)"; h "Current hysteresis bandwidth (A)"
      mask help: This block implements a vector controller.
      mask init:
      | [X1,X1m,X2,X2m,X3,X4,Y1,Y1m,Y2,Y2m,Y3,Y4,color1,color2]=spsdrivelogo;
      mask Display:
      | patch([X1 X1m],[Y1 Y1m],color1);
      | patch(X3,Y3,color2);
      | plot([X1 X1m X2 X2m X3 X4],[Y1 Y1m Y2 Y2m Y3 Y4]);
  + : PMIOPort  Port=1  Side=Left
  - : PMIOPort  Port=2  Side=Left
  Generator : Outport
  Ctrl : Outport  Port=2
  Tem : Outport  Port=3
  wires:
  Enable/1 -> VECT/1(En), Speed Controller/3(En)
  Torque/1 -> Speed Controller/2(N*)
  Speed Controller/1(Torque*) -> VECT/2(Torque*)
  Bus Selector/1 -> Speed Controller/1(N)  "<Rotor speed wm (rad/s)>"
  PMSM1/1 -> Mux/2(m), Bus Selector/1, Generator/1
  Speed (rad/s)/1 -> PMSM1/1
  Bus Selector/3 -> Tem/1  "<Electromagnetic torque Te (N*m)>"
  Measures/1 -> VECT/4(I_abc)
  Speed Controller/2(Ctrl) -> Ctrl/1
  VECT/1(sig*) -> Mux/1(sig*)
  Mux/1(Ctrl) -> Three-phase Inverter/1(ctrl)
  Bus Selector/2 -> VECT/3(teta)  "<Rotor angle thetam (rad)>"
  connections:
  -/RConn1 -- Three-phase Inverter/RConn2
  +/RConn1 -- Three-phase Inverter/RConn1
  Measures/RConn1 -- PMSM1/LConn1
  Measures/RConn2 -- PMSM1/LConn2
  Measures/RConn3 -- PMSM1/LConn3
  Three-phase Inverter/LConn1 -- Measures/LConn1
  Measures/LConn2 -- Three-phase Inverter/LConn2
  Three-phase Inverter/LConn3 -- Measures/LConn3

== system HEV/Electric Motor Controller /Measurements1 ==
  Current : powerlib/Measurements/Current Measurement  PhasorSimulation=off  OutputType=Complex  PSBequivalent=0
  Voltage : powerlib/Measurements/Voltage Measurement  PhasorSimulation=off  OutputType=Complex  PSBequivalent=0
  ideal current ref : PMIOPort  Port=1  Side=Right
  + : PMIOPort  Tag=PMCPort  Port=2  Side=Left
  - : PMIOPort  Port=3  Side=Left
  " ideal current " : Outport
  voltage out : Outport  Port=2
  wires:
  Voltage/1 -> voltage out/1
  Current/1 -> " ideal current "/1
  connections:
  -/RConn1 -- Voltage/LConn2
  ideal current ref/RConn1 -- Current/RConn1
  Current/LConn1 -- Voltage/LConn1 -- +/RConn1

== system HEV/Electric Motor Controller /Measurements2 ==
  Battery : Inport
  Ideal Current Motor : Inport  Port=2
  Voltage : Inport  Port=3
  Ideal Current Generator : Inport  Port=4
  Bus Selector1 : BusSelector  OutputSignals=SOC (%),Current (A),Voltage (V)
  Mux3 : Mux  Inputs=3
  Mux4 : Mux  Inputs=3
  Mux5 : Mux  Inputs=2
  Product1 : Product  RndMeth=Zero
  Product2 : Product  RndMeth=Zero
  Product3 : Product  RndMeth=Zero
  Scope : Scope  NumInputPorts=3
      settings: YMin=-25~0~39.262  YMax=225~225~39.273  SaveName=ScopeData2
  tag scope: Power=global
  wires:
  Battery/1 -> Bus Selector1/1
  Bus Selector1/1 -> Scope/3  "<SOC (%)>"
  Bus Selector1/2 -> Product3/1, Mux4/3  "<Current (A)>"
  Bus Selector1/3 -> Mux5/2, Product3/2  "<Voltage (V)>"
  Product3/1 -> Mux3/3  "Battery Power (W)"
  Ideal Current Motor/1 -> Mux4/1, Product1/1
  Voltage/1 -> Product1/2, Product2/2, Mux5/1
  Product1/1 -> Mux3/1  "Motor Power (W)"
  Ideal Current Generator/1 -> Mux4/2, Product2/1
  Product2/1 -> Mux3/2  "Generator Power (W)"
  Mux4/1 -> Scope/1  "Current (Motor + Generator + Battery)"
  Mux5/1 -> Scope/2  "Voltage ( DC Bus + Battery)"
  Mux3/1 -> [Power]

== system HEV/Electric Motor Controller /Motor 50kW ==
  Enable : Inport
  Torque : Inport  Port=2
  Speed (rad/s) : Inport  Port=3
  500 VDC 50kW PMSM : powerlib/Machines/Permanent Magnet Synchronous Machine  NbPhases=3  FluxDistribution=Sinusoidal  RotorType=Salient-pole  MechanicalLoad=Speed w  PresetModel=No  ShowDetailedParameters=on  MeasurementBus=off  Resistance=0.0065  Inductance=0  dqInductances="[0.001597972349731   0.002057052250467]"  La=0.000835  MachineConstant=Flux linkage established by magnets (V.s)  Flux=0.175666143629361  VoltageCst=127.4493  TorqueCst=1.054  Flat=0  Mechanical=[0.089 0.005 4]  PolePairs=4  InitialConditions=[0,0,0,0]  InitialConditions5ph=[0 0 0 0 0 0]  TsPowergui=0  TsBlock=-1  RefAngle=90 degrees behind phase A axis (modified Park)
      settings: AttributesFormatString=\n
  Bus Selector : BusSelector  OutputSignals=Rotor speed wm (rad/s),Rotor angle thetam (rad),Electromagnetic torque Te (N*m)
  Display : Display
      settings: Decimation=100
  Display1 : Display
      settings: Decimation=100
  Measures : electricdrivelib/AC drives/PM Synchronous Motor Drive/Measures
  Mux : Subsystem
  Speed Controller : Subsystem  mask(Speed controller){SwK=Torque regulation, bs=3000, ramp=[-10000,10000], kp=1/5, ki=50/5, fc=1000/10, ctrl_sat=[-400,400], Tsc=120e-6}
      mask prompts: SwK "Regulation type"; bs "Base speed (rpm)"; ramp "Speed reference ramp (rpm/s) [deceleration,acceleration]"; kp "Proportional gain"; ki "Integral gain"; fc "Speed measurement - low-pass filter cutoff frequency (Hz)"; ctrl_sat "Controller output torque saturation (N.m) [negative,positive]"; Tsc "Controller sampling time (s)"
      mask help: This block implements a PI speed regulator.
      mask init:
      | [X1,X1m,X2,X2m,X3,X4,Y1,Y1m,Y2,Y2m,Y3,Y4,color1,color2]=spsdrivelogo;
      mask TypeOptions SwK: Speed regulation | Torque regulation
      mask Display:
      | patch([X1 X1m],[Y1 Y1m],color1);
      | patch(X3,Y3,color2);
      | plot([X1 X1m X2 X2m X3 X4],[Y1 Y1m Y2 Y2m Y3 Y4]);
  Three-phase Inverter : Subsystem  mask(SPSdrives Converter){Arms=3, SnubberResistance=5000, SnubberCapacitance=inf, Device=IGBT / Diodes, Ron=1e-3, Lon=0, ForwardVoltages=[0.8,0.8], ForwardVoltage=0, GTOparameters=[0,0], IGBTparameters=[1e-6,2e-6], Measurements=All voltages and currents, SourceFrequency=60, dqInductances=[0.001597972349731   0.002057052250467], Flux=0.175666143629361, Resistance=0.0065, p=4, converterType=Inverter}
      mask prompts: Arms "Number of bridge arms:"; SnubberResistance "Snubber resistance Rs (Ohms)"; SnubberCapacitance "Snubber capacitance Cs (F)"; Device "Power Electronic device"; Ron "Ron (Ohms)"; Lon "Lon (H)"; ForwardVoltages "Forward voltages  [ Device Vf(V) , Diode Vfd(V)]"; ForwardVoltage "Forward voltage Vf (V)"; GTOparameters "[  Tf (s) , Tt (s)  ]"; IGBTparameters "[  Tf (s) , Tt (s)  ]"; SourceFrequency "Source Frequency (Hz)"; dqInductances "PMSM-Inductances [ Ld(H) Lq(H) ]:"; Flux "PMSM-Flux induced by magnets (Wb):"; Resistance "PMSM-Stator resistance Rs (ohm):"; p "PMSM-Pairs of poles p:"; converterType "Converter type:"
      mask init:
      | Ld=dqInductances(1);
      | Lq=dqInductances(2);
      | Fcs=6*SourceFrequency/10;
      settings: OpenFcn=power_openblockproxy();
      mask Help: web(psbhelp);
      mask TypeOptions Arms: 1 | 2 | 3
      mask TypeOptions Device: Diodes | Thyristors | GTO / Diodes | MOSFET / Diodes | IGBT / Diodes | Ideal Switches
      mask TypeOptions Measurements: None | Device voltages | Device currents | UAB UBC UCA UDC voltages | All voltages and currents
      mask TypeOptions converterType: Rectifier | Inverter
      mask Display: plot(0,0,100,100,[39 39 23.8],[71 28 28],[44 56 49.6 56 52.8 56 61 61],[39.2 33.6 32.8 33.6 40.8 33.6 30 12.4],[44 44 44 61 61],[28 71 60 66.4 90],[75 67 83 75 67 83 75 75],[54 42 42 54 54 54 54 66],[61 75 75],[24 24 42],[75 75 61],[66,76,76])
  Torque limitation : Subsystem
      mask Display: plot([0;1800;2000;2500;3000;3500], [1;1;0.90*1;0.72*1;0.6*1;0.51*1])
  VECT controller : Subsystem  mask(VECT){nb_p=4, dqInductances=[0.001597972349731   0.002057052250467], lambda=0.175666143629361, Ts_vect=60e-6}
      mask prompts: nb_p "Motor pairs of poles"; dqInductances "Inductances [ Ld(H) Lq(H) ]:"; lambda "Flux induced by magnets (Wb)"; Ts_vect "Sampling time (s)"
      mask help: This block implements a vector controller.
      mask init:
      | [X1,X1m,X2,X2m,X3,X4,Y1,Y1m,Y2,Y2m,Y3,Y4,color1,color2]=spsdrivelogo;
      | ib = lambda/(dqInductances(2)-dqInductances(1));
      | Teb = 3/2*nb_p*lambda*ib;
      | Ld = dqInductances(1);
      | Lq = dqInductances(2);
      | lam = lambda;
      | p=nb_p;
      | ib = lam/(Lq-Ld);
      | iqn = 0:0.01:3;
      | ten = iqn/2.*(sqrt(4*iqn.*iqn+1)+1);
      mask Display:
      | patch([X1 X1m],[Y1 Y1m],color1);
      | patch(X3,Y3,color2);
      | plot([X1 X1m X2 X2m X3 X4],[Y1 Y1m Y2 Y2m Y3 Y4]);
  + : PMIOPort  Port=1  Side=Left
  - : PMIOPort  Port=2  Side=Left
  Motor : Outport
  Ctrl : Outport  Port=2
  Tem : Outport  Port=3
  wires:
  Mux/1(Ctrl) -> Three-phase Inverter/1(ctrl)
  VECT controller/1(sig*) -> Mux/1(sig)
  Speed Controller/2(Ctrl) -> Ctrl/1
  Speed (rad/s)/1 -> Display1/1, 500 VDC 50kW PMSM/1
  500 VDC 50kW PMSM/1 -> Bus Selector/1, Mux/2(m), Motor/1
  Bus Selector/3 -> Tem/1  "<Electromagnetic torque Te (N*m)>"
  Bus Selector/1 -> VECT controller/3(w), Speed Controller/1(N), Torque limitation/1(N rad/s)  "<Rotor speed wm (rad/s)>"
  Enable/1 -> VECT controller/1(En), Speed Controller/3(En)
  Speed Controller/1(Torque*) -> Display/1, VECT controller/2(Torque*)
  Measures/1 -> VECT controller/5(I_abc)
  Bus Selector/2 -> VECT controller/4(teta)  "<Rotor angle thetam (rad)>"
  Torque limitation/1(torque) -> Speed Controller/2(N*)
  Torque/1 -> Torque limitation/2(Torque)
  connections:
  Three-phase Inverter/LConn3 -- Measures/LConn3
  Measures/LConn2 -- Three-phase Inverter/LConn2
  Three-phase Inverter/LConn1 -- Measures/LConn1
  Measures/RConn3 -- 500 VDC 50kW PMSM/LConn3
  Measures/RConn2 -- 500 VDC 50kW PMSM/LConn2
  Measures/RConn1 -- 500 VDC 50kW PMSM/LConn1
  +/RConn1 -- Three-phase Inverter/RConn1
  -/RConn1 -- Three-phase Inverter/RConn2

== system HEV/Electric Motor Controller /demux ==
  motor : Inport
  Ctrl : Inport  Port=2
  "+ -> -1" : Gain  Gain=30/pi
  Bus Selector : BusSelector  OutputSignals=Stator current is_a (A),Rotor speed wm (rad/s),Electromagnetic torque Te (N*m)
  Bus Selector1 : BusSelector  OutputSignals=Torque reference (Nm)
  Mux1 : Mux  Inputs=2
  Product : Product  RndMeth=Zero
  i_a : Outport
  speed : Outport  Port=2
  Torque : Outport  Port=3
  Power : Outport  Port=4
  wires:
  "+ -> -1"/1 -> speed/1
  motor/1 -> Bus Selector/1
  Ctrl/1 -> Bus Selector1/1
  Bus Selector/2 -> Product/2, "+ -> -1"/1  "<Rotor speed wm (rad/s)>"
  Bus Selector/3 -> Mux1/1, Product/1  "<Electromagnetic torque Te (N*m)>"
  Bus Selector1/1 -> Mux1/2  "<Torque reference (Nm)>"
  Mux1/1 -> Torque/1
  Bus Selector/1 -> i_a/1  "<Stator current is_a (A)>"
  Product/1 -> Power/1

== system HEV/Electric Motor Controller /demux Gen ==
  Generator : Inport
  Ctrl : Inport  Port=2
  "+ -> -1" : Gain  Gain=30/pi
  Bus Selector : BusSelector  OutputSignals=Stator current is_a (A),Rotor speed wm (rad/s),Electromagnetic torque Te (N*m)
  Bus Selector1 : BusSelector  OutputSignals=Torque reference (Nm)
  Mux1 : Mux  Inputs=2
  Product : Product  RndMeth=Zero
  Current : Outport
  Speed : Outport  Port=2
  Torque : Outport  Port=3
  Power : Outport  Port=4
  wires:
  "+ -> -1"/1 -> Speed/1
  Generator/1 -> Bus Selector/1
  Ctrl/1 -> Bus Selector1/1
  Bus Selector/2 -> Product/2, "+ -> -1"/1  "<Rotor speed wm (rad/s)>"
  Bus Selector/3 -> Product/1, Mux1/1  "<Electromagnetic torque Te (N*m)>"
  Bus Selector1/1 -> Mux1/2  "<Torque reference (Nm)>"
  Mux1/1 -> Torque/1
  Bus Selector/1 -> Current/1  "<Stator current is_a (A)>"
  Product/1 -> Power/1

== system HEV/Engine Controller/Fuel and Gas Emissions Calculation ==
  Engine speed (rpm) : Inport
  Torque (Nm) : Inport  Port=2
  Add : Sum
  CO Emissions Table : Lookup2D  RowIndex=GasEmisTable.speed  ColumnIndex=GasEmisTable.torque  Table=GasEmisTable.lookupTableCO
  Constant : Constant  Value=final_fuelConsumed(end)
  Fuel Consumption Table : Lookup2D  RowIndex=FuelConsTable.speed  ColumnIndex=FuelConsTable.torque  Table=FuelConsTable.lookupTableFuel
  Fuel Conversion : Subsystem
  HC Emissions Table : Lookup2D  RowIndex=GasEmisTable.speed  ColumnIndex=GasEmisTable.torque  Table=GasEmisTable.lookupTableHC
  NOX Emissions Table : Lookup2D  RowIndex=GasEmisTable.speed  ColumnIndex=GasEmisTable.torque  Table=GasEmisTable.lookupTableNOX
  total fuel (L) : Display
      settings: Decimation=100
  Fuel (L/100km) : Outport
  CO Emissions (g/s) : Outport  Port=2
  HC Emissions (g/s) : Outport  Port=3
  NOX Emissions (g/s) : Outport  Port=4
  Total Fuel (L) : Outport  Port=5
  wires:
  Fuel Conversion/3(Total Fuel (l)) -> Add/1
  Fuel Consumption Table/1 -> Fuel Conversion/2(Fuel Consumption (g/s))  "Fuel Consumption (g/s)"
  Fuel Conversion/1(l/100km) -> Fuel (L/100km)/1
  [VehSpeed_kmh] -> Fuel Conversion/1(Vehicle Speed (km/h))
  Torque (Nm)/1 -> Fuel Consumption Table/2, CO Emissions Table/2, HC Emissions Table/2, NOX Emissions Table/2
  Engine speed (rpm)/1 -> Fuel Consumption Table/1, NOX Emissions Table/1, HC Emissions Table/1, CO Emissions Table/1
  HC Emissions Table/1 -> HC Emissions (g/s)/1
  NOX Emissions Table/1 -> NOX Emissions (g/s)/1
  CO Emissions Table/1 -> CO Emissions (g/s)/1
  Constant/1 -> Add/2
  Add/1 -> total fuel (L)/1, Total Fuel (L)/1

== system HEV/Engine Controller/Gasoline Engine ==
  note: The throttle signal value indicates the torque demand
      | relative to maximum available torque. If the engine
      | speed rises above the maximum allowed, the output
      | torque is cut to zero. Saturation is applied to keep the
      | throttle signal between zero and one.
      |
      | The air-fuel combustion dynamics is not modeled.
  Throttle : Inport
  Compare To Constant : simulink/Logic and Bit Operations/Compare To Constant  relop=>  const=speed_max*2*pi/60  OutDataTypeStr=uint8  ZeroCross=off
  Constant : Constant  Value=0
  Engine Speed Assertion : Assertion  AssertionFailFcn=disp('Engine speed (rpm) exceeded maximum speed during the simulation. Simulation results could be inaccurate or unpredictable.')  StopWhenAssertionFail=off
  Gain : Gain  Gain=60/(2*pi)
  Logical Operator : Logic  Operator=NOT  AllPortsSameDT=off  OutDataTypeStr=boolean
  Motion Sensor : driveline/Sensors & Actuators/Motion Sensor  Angle=off  x0=5  Velocity=on  Acceleration=off
  Peak torque : Lookup  InputValues=speed  Table=torque  SaturateOnIntegerOverflow=on
  Product : Product  SaturateOnIntegerOverflow=on  OutDataTypeStr=Inherit: Same as first input
  Saturation : Saturate  UpperLimit=1.0  LowerLimit=0.0
  Saturation1 : Saturate  UpperLimit=6000*pi/30  LowerLimit=0
  Saturation2 : Saturate  UpperLimit=136  LowerLimit=0
  Switch : Switch  Threshold=1
  Torque Actuator : driveline/Sensors & Actuators/Torque Actuator
  Connection Port : PMIOPort  Port=1  Side=Right
  wires:
  Saturation/1 -> Product/2
  Throttle/1 -> Saturation/1
  Constant/1 -> Switch/1
  Compare To Constant/1 -> Switch/2, Logical Operator/1
  Product/1 -> Saturation2/1
  Motion Sensor/1 -> Saturation1/1, Gain/1
  Gain/1 -> Peak torque/1
  Peak torque/1 -> Product/1
  Logical Operator/1 -> Engine Speed Assertion/1
  Saturation1/1 -> Compare To Constant/1
  Switch/1 -> Torque Actuator/1
  Saturation2/1 -> Switch/3
  connections:
  Connection Port/RConn1 -- Torque Actuator/RConn1 -- Motion Sensor/LConn1

== system HEV/Power Controller/Battery Management System ==
  Batt : Inport
  Battery discharge range : Saturate  UpperLimit=21000  LowerLimit=0
  Battery maximum power : Gain  Gain=-21000
  Bus Selector : BusSelector  OutputSignals=Voltage (V),SOC (%)
  Compare To Constant1 : simulink/Logic and Bit Operations/Compare To Constant  relop=<  const=30  OutDataTypeStr=boolean
  Compare To Constant2 : simulink/Logic and Bit Operations/Compare To Constant  relop=>  const=80  OutDataTypeStr=boolean
  Data Type Conversion : DataTypeConversion  OutDataTypeStr=double  SampleTime=0
  Data Type Conversion1 : DataTypeConversion  OutDataTypeStr=double  SampleTime=0
  Nominal power : Constant  Value=21000
  Nominal voltage : Constant  Value=100
  Rate Limiter : RateLimiter  RisingSlewLimit=21000*2  FallingSlewLimit=-21000*2  SampleTimeMode=inherited
  Rate Limiter1 : RateLimiter  RisingSlewLimit=21000*10  FallingSlewLimit=-21000*10  SampleTimeMode=inherited
  S-R Flip-Flop : simulink_extras/Flip Flops/S-R Flip-Flop  initial_condition=0
  Sum1 : Sum  Inputs=+-|
  Sum2 : Sum  Inputs=+-|
  Terminator : Terminator
  V2W : Gain  Gain=200
  Battery power : Outport
  Battery limit : Outport  Port=2
  wires:
  Batt/1 -> Bus Selector/1
  Battery maximum power/1 -> Rate Limiter/1
  S-R Flip-Flop/2 -> Terminator/1
  Bus Selector/2 -> Compare To Constant1/1, Compare To Constant2/1  "<SOC (%)>"
  Data Type Conversion/1 -> Battery maximum power/1
  Compare To Constant1/1 -> S-R Flip-Flop/1
  Compare To Constant2/1 -> S-R Flip-Flop/2
  S-R Flip-Flop/1 -> Data Type Conversion/1
  Sum2/1 -> V2W/1
  V2W/1 -> Sum1/2
  Nominal power/1 -> Sum1/1
  Sum1/1 -> Data Type Conversion1/1
  Data Type Conversion1/1 -> Battery discharge range/1
  Battery discharge range/1 -> Rate Limiter1/1
  Bus Selector/1 -> Sum2/2  "<Voltage (V)>"
  Nominal voltage/1 -> Sum2/1
  Rate Limiter1/1 -> Battery limit/1
  Rate Limiter/1 -> Battery power/1

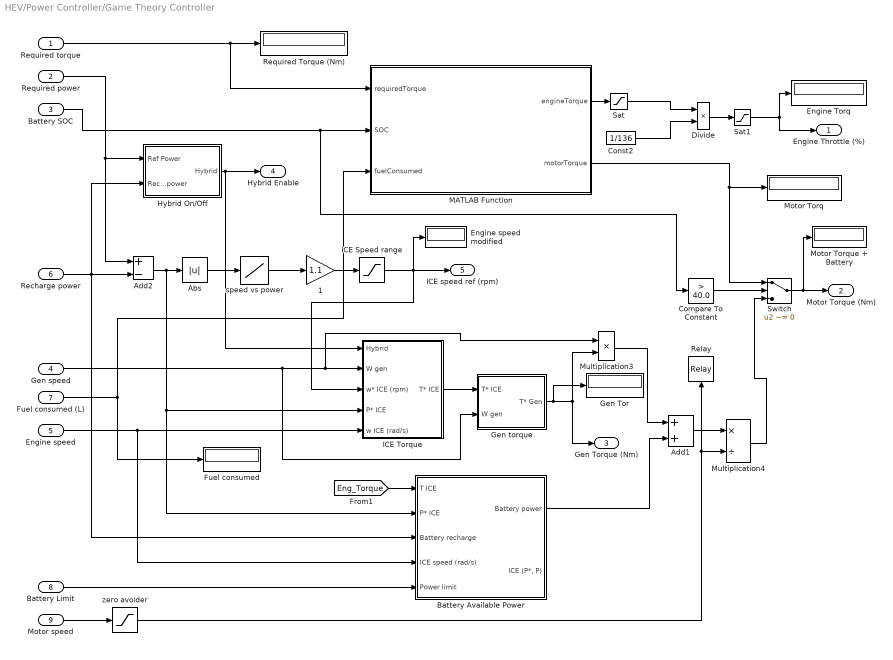
== system HEV/Power Controller/Game Theory Controller ==
  Required torque : Inport  OutDataTypeStr=double  PortDimensions=1
  Required power : Inport  Port=2
  Battery SOC : Inport  Port=3
  Gen speed : Inport  Port=4
  Engine speed : Inport  Port=5
  Recharge power : Inport  Port=6
  Fuel consumed (L) : Inport  Port=7
  Battery Limit : Inport  Port=8
  Motor speed : Inport  Port=9
  " 1" : Gain  Gain=1.1
  Abs : Abs
  Add1 : Sum
  Add2 : Sum  Inputs=+-
  Battery Available Power : Subsystem
  Compare To Constant : simulink/Logic and Bit Operations/Compare To Constant  relop=>  const=40.0  OutDataTypeStr=uint8
  Const2 : Constant  Value=1/136
  Divide : Product  Inputs=**
  Engine Torq : Display
      settings: Decimation=100
  Engine speed modified : Display
      settings: Decimation=100
  Fuel consumed : Display
      settings: Decimation=100
  Gen Tor : Display
      settings: Decimation=100
  Gen torque : Subsystem
  Hybrid On/Off : Subsystem
  ICE Speed range : Saturate  UpperLimit=5000  LowerLimit=750
  ICE Torque : Subsystem
  MATLAB Function : MATLAB Function  TreatAsAtomicUnit=on
  Motor Torq : Display
      settings: Decimation=100
  Motor Torque + Battery : Display
      settings: Decimation=100
  Multiplication3 : Product
  Multiplication4 : Product  Inputs=*/
  Relay : Relay  OnSwitchValue=200/30*pi  OffSwitchValue=100/30*pi  OnOutputValue=0  OffOutputValue=1
  Required Torque (Nm) : Display
      settings: Decimation=100
  Sat : Saturate  UpperLimit=136  LowerLimit=0
  Sat1 : Saturate  UpperLimit=1  LowerLimit=0
  Switch : Switch  Criteria=u2 ~= 0
  speed vs power : Lookup  InputValues=EngineSpeedPower.power  Table=EngineSpeedPower.speed  SaturateOnIntegerOverflow=on
  zero avoider : Saturate  UpperLimit=inf  LowerLimit=1
  Engine Throttle (%) : Outport
  Motor Torque (Nm) : Outport  Port=2
  Gen Torque (Nm) : Outport  Port=3
  Hybrid Enable : Outport  Port=4
  ICE speed ref (rpm) : Outport  Port=5
  wires:
  Required torque/1 -> MATLAB Function/1(requiredTorque), Required Torque (Nm)/1
  Battery SOC/1 -> Compare To Constant/1, MATLAB Function/2(SOC)
  Required power/1 -> Add2/1, Hybrid On/Off/1(Ref Power)
  Recharge power/1 -> Battery Available Power/3(Battery recharge), Add2/2, Hybrid On/Off/2(Recharge power)
  Add2/1 -> Battery Available Power/2(P* ICE), ICE Torque/4(P* ICE), Abs/1
  Abs/1 -> speed vs power/1
  speed vs power/1 -> " 1"/1
  " 1"/1 -> ICE Speed range/1
  ICE Speed range/1 -> ICE Torque/3(w* ICE (rpm)), ICE speed ref (rpm)/1, Engine speed modified/1
  Hybrid On/Off/1(Hybrid) -> Hybrid Enable/1, ICE Torque/1(Hybrid)
  Engine speed/1 -> Battery Available Power/4(ICE speed (rad/s)), ICE Torque/5(w ICE (rad/s))
  ICE Torque/1(T* ICE) -> Gen torque/1(T* ICE)
  MATLAB Function/1(engineTorque) -> Sat/1
  Fuel consumed (L)/1 -> MATLAB Function/3(fuelConsumed), Fuel consumed/1
  MATLAB Function/2(motorTorque) -> Switch/1, Motor Torq/1
  Gen torque/1(T* Gen) -> Gen Torque (Nm)/1, Multiplication3/2, Gen Tor/1
  Sat/1 -> Divide/1
  Const2/1 -> Divide/2
  Divide/1 -> Sat1/1
  Sat1/1 -> Engine Throttle (%)/1, Engine Torq/1
  [Eng_Torque] -> Battery Available Power/1(T ICE)
  Battery Limit/1 -> Battery Available Power/5(Power limit)
  Motor speed/1 -> zero avoider/1
  zero avoider/1 -> Multiplication4/2, Relay/1
  Gen speed/1 -> Gen torque/2(W gen), Multiplication3/1, ICE Torque/2(W gen)
  Multiplication3/1 -> Add1/1
  Battery Available Power/1(Battery power) -> Add1/2
  Add1/1 -> Multiplication4/1
  Multiplication4/1 -> Switch/3
  Switch/1 -> Motor Torque + Battery/1, Motor Torque (Nm)/1
  Compare To Constant/1 -> Switch/2
